simulink model "MPSK_passmodem_v2"  (Simulink 7.6)
settings: Solver=FixedStepDiscrete  SolverMode=SingleTasking  StartTime=0.0  StopTime=1  FixedStep=1/100000  RelTol=1e-3  AbsTol=1e-6
PreLoadFcn:
  | fs=1e5; Ts=1/fs; R=1000; T=1/R; fc=10000; M=8; offset=0;
undefined symbols (not defined in the file): get
libraries: simulink x10, commfilt2 x6, commsink2 x4, simulink_extras x2, commutil2 x2, commchan3 x1, commrandsrc2 x1
settings Model: Creator=amoura  LastModifiedBy=Sílvio
settings DataIOCC: LimitDataPoints=off
settings OptimizationCC: BlockReduction=off  BooleanDataType=off  InitFltsAndDblsToZero=on
settings DebuggingCC: SaveWithParameterizedLinksMsg=none  SignalResolutionControl=TryResolveAllWithWarning  SolverPrmCheckMsg=none  MultiTaskDSMMsg=warning  MultiTaskCondExecSysMsg=none  StrictBusMsg=None
settings HardwareCC: TargetUnknown=on
settings RTWCC: TemplateMakefile=grt_unix.tmf  IncludeERTFirstTime=on
settings GRTTargetCC: TargetFcnLib=ansi_tfl_tmw.mat  ModelReferenceCompliant=off  MatFileLogging=off

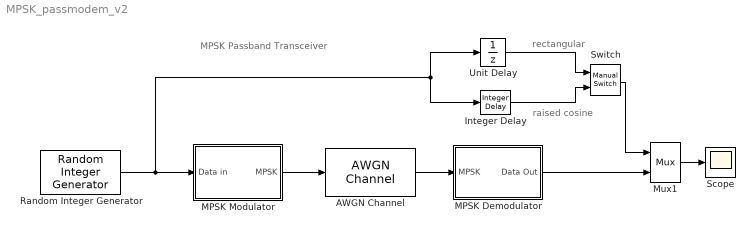
== system MPSK_passmodem_v2 ==
  note: raised cosine
  note: rectangular
  note: MPSK Passband Transceiver
  AWGN Channel : commchan3/AWGN Channel  SystemSampleTime=-1  InputProcessing=Columns as channels (frame based)  seed=67  noiseMode="Signal to noise ratio  (Es/No)"  EbNodB=0  EsNodB=100  SNRdB=10  bitsPerSym=1  Ps=1  Tsym=T  variance=0.1
  Integer Delay : simulink/Discrete/Integer Delay  NumDelays=2*5  vinit=0  samptime=-1
  MPSK Demodulator : Subsystem
  MPSK Modulator : Subsystem
  Mux1 : Mux  Inputs=2
  Random Integer Generator : commrandsrc2/Random Integer Generator  SystemSampleTime=-1  mul=M  seed=96931  Ts=T  frameBased=off  sampPerFrame=100  orient=off  outDataType=double
  Scope : Scope
      settings: TickLabels=on  YMin=-1  YMax=8  DataFormat=Array
  Switch : simulink/Signal Routing/Manual Switch  SystemSampleTime=-1  sw=0  action=0  varsize=off
  Unit Delay : UnitDelay  SampleTime=T
  wires:
  MPSK Modulator/1(MPSK) -> AWGN Channel/1
  Mux1/1 -> Scope/1
  Random Integer Generator/1 -> MPSK Modulator/1(Data in), Unit Delay/1, Integer Delay/1
  MPSK Demodulator/1(Data Out) -> Mux1/2
  AWGN Channel/1 -> MPSK Demodulator/1(MPSK)
  Integer Delay/1 -> Switch/2
  Unit Delay/1 -> Switch/1
  Switch/1 -> Mux1/1

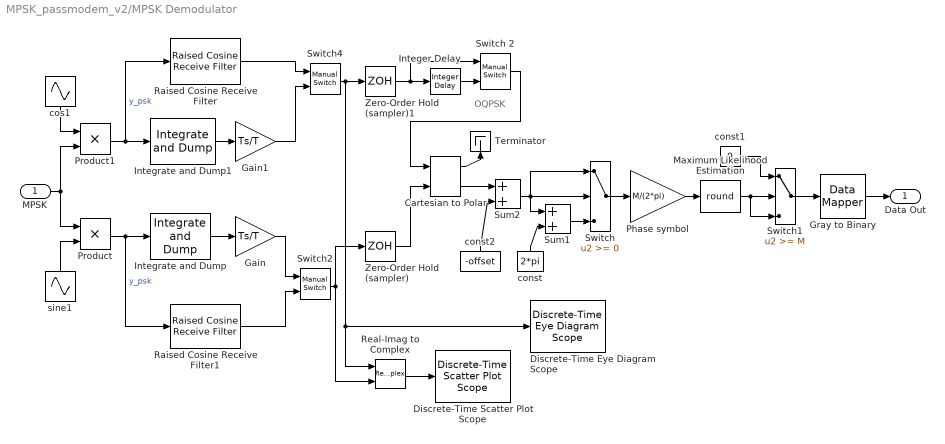
== system MPSK_passmodem_v2/MPSK Demodulator ==
  note: OQPSK
  MPSK : Inport
  Cartesian to Polar : simulink_extras/Transformations/Cartesian to Polar  SystemSampleTime=-1
  Discrete-Time Eye Diagram Scope : commsink2/Discrete-Time Eye Diagram Scope  Tag=EyeDiagram  SystemSampleTime=-1  sampPerSymb=100  offsetEye=0  symbPerTrace=2  numTraces=100  numNewFrames=4  LineStyles=-  LineColors=b  dupPoints=on  fading=on  render=on  AxisGrid=on  yMin=-0.707831262397474  yMax=0.776216891487404  inphaseLabel=In-phase Amplitude  quadratureLabel=Quadrature Amplitude  openScopeAtSimStart=on  dispDiagram=In-phase Only  FrameNumber=off  FigPos=get(0,'defaultfigureposition');  figTitle=Receiver In-Phase Eye Diagram  block_type_=eye  numLinesMax=8
  Discrete-Time Scatter Plot Scope : commsink2/Discrete-Time Scatter Plot Scope  Tag=ScatterPlot  SystemSampleTime=-1  sampPerSymb=fs/R  offsetEye=0  numTraces=40  numNewFrames=10  LineMarkers=.  LineColors=b  fading=on  render=on  AxisGrid=on  xMin=-0.526661007972348  xMax=0.526437343582541  yMin=-0.52656219857096  yMax=0.526536152983929  inphaseLabel=In-phase Amplitude  quadratureLabel=Quadrature Amplitude  openScopeAtSimStart=on  FrameNumber=off  FigPos=get(0,'defaultfigureposition');  figTitle=Receiver Scatter Plot  numLinesMax=8  block_type_=scatter
  Gain : Gain  Gain=Ts/T  SampleTime=Ts  SaturateOnIntegerOverflow=on  OutDataTypeStr=Inherit: Same as input  ParamDataTypeStr=Inherit: Same as input
  Gain1 : Gain  Gain=Ts/T  SampleTime=Ts  SaturateOnIntegerOverflow=on  OutDataTypeStr=Inherit: Same as input  ParamDataTypeStr=Inherit: Same as input
  Gray to Binary : commutil2/Data Mapper  SystemSampleTime=-1  MapMode=Gray to Binary  M=M  MapVec=[0 1 3 2 7 6 4 5]
  Integer Delay : simulink/Discrete/Integer Delay  NumDelays=(T/Ts)/2  vinit=0  samptime=-1
  Integrate and Dump : commfilt2/Integrate and Dump  DialogController=commDDGCreate  DialogControllerArgs=DataTag3  obssamples=T/Ts  offsetsamples=1  nodump=on  roundingMode=Floor  overflowMode=off
  Integrate and Dump1 : commfilt2/Integrate and Dump  DialogController=commDDGCreate  DialogControllerArgs=DataTag4  obssamples=T/Ts  offsetsamples=1  nodump=on  roundingMode=Floor  overflowMode=off
  Maximum Likelihood Estimation : Rounding  Operator=round
  Phase symbol : Gain  Gain=M/(2*pi)  SaturateOnIntegerOverflow=on  OutDataTypeStr=Inherit: Same as input  ParamDataTypeStr=Inherit: Same as input
  Product : Product  SampleTime=1/100000  SaturateOnIntegerOverflow=on  RndMeth=Zero  InputSameDT=on  OutDataTypeStr=Inherit: Same as first input
  Product1 : Product  SampleTime=1/100000  SaturateOnIntegerOverflow=on  RndMeth=Zero  InputSameDT=on  OutDataTypeStr=Inherit: Same as first input
  Raised Cosine Receive Filter : commfilt2/Raised Cosine Receive Filter  DialogController=dspDDGCreate  DialogControllerArgs=DataTag6  SystemSampleTime=-1  filtType=Normal  N=100  D=5  R=0.4  sampMode=Mute  saveAsFlag=0  rateMode=None  downFactor=100  downOffset=0  framing=Enforce single-rate processing  InputProcessing=Columns as channels (frame based)  checkGain=Normalized  filterGain=1  checkCoeff=off  variableName=rcRxFilt  launchFVT=off  roundingMode=Floor  overflowMode=off
  Raised Cosine Receive Filter1 : commfilt2/Raised Cosine Receive Filter  DialogController=dspDDGCreate  DialogControllerArgs=DataTag8  SystemSampleTime=-1  filtType=Normal  N=100  D=5  R=0.4  sampMode=Mute  saveAsFlag=0  rateMode=None  downFactor=100  downOffset=0  framing=Enforce single-rate processing  InputProcessing=Columns as channels (frame based)  checkGain=Normalized  filterGain=1  checkCoeff=off  variableName=rcRxFilt1  launchFVT=off  roundingMode=Floor  overflowMode=off
  Real-Imag to Complex : RealImagToComplex
  Sum1 : Sum  SaturateOnIntegerOverflow=on  InputSameDT=on  OutDataTypeStr=Inherit: Same as first input
  Sum2 : Sum  SaturateOnIntegerOverflow=on  InputSameDT=on  OutDataTypeStr=Inherit: Same as first input
  Switch : Switch  SaturateOnIntegerOverflow=on  InputSameDT=on
  Switch 2 : simulink/Signal Routing/Manual Switch  SystemSampleTime=-1  sw=1  action=0  varsize=off
  Switch1 : Switch  Threshold=M
  Switch2 : simulink/Signal Routing/Manual Switch  SystemSampleTime=-1  sw=1  action=0  varsize=off
  Switch4 : simulink/Signal Routing/Manual Switch  SystemSampleTime=-1  sw=0  action=0  varsize=off
  Terminator : Terminator
  Zero-Order Hold (sampler) : ZeroOrderHold  SampleTime=T
  Zero-Order Hold (sampler)1 : ZeroOrderHold  SampleTime=T
  const : Constant  Value=2*pi
  const1 : Constant  Value=0
  const2 : Constant  Value=-offset
  cos1 : Sin  Frequency=2*pi*fc  Phase=pi/2  SampleTime=0
  sine1 : Sin  Frequency=2*pi*fc  SampleTime=0
  Data Out : Outport
  wires:
  Product/1 -> Raised Cosine Receive Filter1/1, Integrate and Dump/1  "y_psk"
  MPSK/1 -> Product1/2, Product/1
  Integrate and Dump/1 -> Gain/1
  sine1/1 -> Product/2
  Product1/1 -> Integrate and Dump1/1, Raised Cosine Receive Filter/1  "y_psk"
  Integrate and Dump1/1 -> Gain1/1
  cos1/1 -> Product1/1
  Sum1/1 -> Switch/3
  Switch/1 -> Phase symbol/1
  Cartesian to Polar/1 -> Terminator/1
  Phase symbol/1 -> Maximum Likelihood Estimation/1
  Zero-Order Hold (sampler)/1 -> Cartesian to Polar/2
  const/1 -> Sum1/2
  Switch1/1 -> Gray to Binary/1
  Maximum Likelihood Estimation/1 -> Switch1/2, Switch1/3
  const1/1 -> Switch1/1
  Real-Imag to Complex/1 -> Discrete-Time Scatter Plot Scope/1
  Gray to Binary/1 -> Data Out/1
  Sum2/1 -> Switch/2, Switch/1, Sum1/1
  Raised Cosine Receive Filter/1 -> Switch4/1
  Gain1/1 -> Switch4/2
  Switch4/1 -> Zero-Order Hold (sampler)1/1, Discrete-Time Eye Diagram Scope/1, Real-Imag to Complex/1
  Gain/1 -> Switch2/1
  Switch2/1 -> Zero-Order Hold (sampler)/1, Real-Imag to Complex/2
  const2/1 -> Sum2/2
  Cartesian to Polar/2 -> Sum2/1
  Raised Cosine Receive Filter1/1 -> Switch2/2
  Integer Delay/1 -> Switch 2/2
  Zero-Order Hold (sampler)1/1 -> Integer Delay/1, Switch 2/1
  Switch 2/1 -> Cartesian to Polar/1

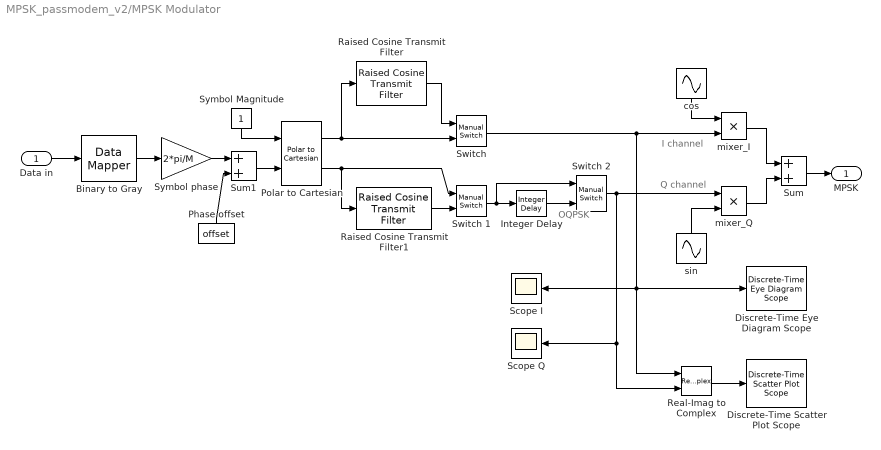
== system MPSK_passmodem_v2/MPSK Modulator ==
  note: I channel
  note: Q channel
  note: OQPSK
  Data in : Inport
  Binary to Gray : commutil2/Data Mapper  SystemSampleTime=-1  MapMode=Binary to Gray  M=M  MapVec=[0 1 3 2 7 6 4 5]
  Discrete-Time Eye Diagram Scope : commsink2/Discrete-Time Eye Diagram Scope  Tag=EyeDiagram  SystemSampleTime=-1  sampPerSymb=100  offsetEye=0  symbPerTrace=2  numTraces=100  numNewFrames=4  LineStyles=-  LineColors=b  dupPoints=on  fading=on  render=on  AxisGrid=on  yMin=-0.141806551380073  yMax=0.145121518302209  inphaseLabel=In-phase Amplitude  quadratureLabel=Quadrature Amplitude  openScopeAtSimStart=on  dispDiagram=In-phase Only  FrameNumber=off  FigPos=get(0,'defaultfigureposition');  figTitle=Transmitter In-Phase Eye Diagram  block_type_=eye  numLinesMax=8
  Discrete-Time Scatter Plot Scope : commsink2/Discrete-Time Scatter Plot Scope  Tag=ScatterPlot  SystemSampleTime=-1  sampPerSymb=fs/R  offsetEye=0  numTraces=40  numNewFrames=10  LineMarkers=.  LineColors=b  fading=on  render=on  AxisGrid=on  xMin=-0.124708902328642  xMax=0.13818390082743  yMin=-0.133971316328163  yMax=0.128921486827909  inphaseLabel=In-phase Amplitude  quadratureLabel=Quadrature Amplitude  openScopeAtSimStart=on  FrameNumber=off  FigPos=get(0,'defaultfigureposition');  figTitle=Transmitter Scatter Plot  numLinesMax=8  block_type_=scatter
  Integer Delay : simulink/Discrete/Integer Delay  NumDelays=(T/Ts)/2  vinit=0  samptime=-1
  Phase offset : Constant  Value=offset  SampleTime=T
  Polar to Cartesian : simulink_extras/Transformations/Polar to Cartesian  SystemSampleTime=-1
  Raised Cosine Transmit Filter : commfilt2/Raised Cosine Transmit Filter  DialogController=dspDDGCreate  DialogControllerArgs=DataTag11  SystemSampleTime=-1  filtType=Square root  D=5  R=0.4  sampMode=Mute  saveAsFlag=0  N=100  framing=Allow multirate processing  checkGain=Normalized  filterGain=1  checkCoeff=off  variableName=rcTxFilt  launchFVT=off  roundingMode=Floor  overflowMode=off
  Raised Cosine Transmit Filter1 : commfilt2/Raised Cosine Transmit Filter  DialogController=dspDDGCreate  DialogControllerArgs=DataTag13  SystemSampleTime=-1  filtType=Square root  D=5  R=0.4  sampMode=Mute  saveAsFlag=0  N=100  framing=Allow multirate processing  checkGain=Normalized  filterGain=1  checkCoeff=off  variableName=rcTxFilt1  launchFVT=off  roundingMode=Floor  overflowMode=off
  Real-Imag to Complex : RealImagToComplex
  Scope I : Scope
      settings: TickLabels=on  TimeRange=0.01  YMin=-2  YMax=2  DataFormat=Array
  Scope Q : Scope
      settings: TickLabels=on  TimeRange=0.01  YMin=-2  YMax=2  SaveName=ScopeData2  DataFormat=Array
  Sum : Sum  SaturateOnIntegerOverflow=on  InputSameDT=on  OutDataTypeStr=Inherit: Same as first input
  Sum1 : Sum  SaturateOnIntegerOverflow=on  InputSameDT=on  OutDataTypeStr=Inherit: Same as first input
  Switch : simulink/Signal Routing/Manual Switch  SystemSampleTime=-1  sw=1  action=0  varsize=off
  Switch 1 : simulink/Signal Routing/Manual Switch  SystemSampleTime=-1  sw=0  action=0  varsize=off
  Switch 2 : simulink/Signal Routing/Manual Switch  SystemSampleTime=-1  sw=1  action=0  varsize=off
  Symbol Magnitude : Constant  SampleTime=T
  Symbol phase : Gain  Gain=2*pi/M  SaturateOnIntegerOverflow=on  OutDataTypeStr=Inherit: Same as input  ParamDataTypeStr=Inherit: Same as input
  cos : Sin  Frequency=2*pi*fc  Phase=pi/2  SampleTime=0
  mixer_I : Product  SampleTime=Ts  SaturateOnIntegerOverflow=on  InputSameDT=on  OutDataTypeStr=Inherit: Same as first input
  mixer_Q : Product  SampleTime=Ts  SaturateOnIntegerOverflow=on  InputSameDT=on  OutDataTypeStr=Inherit: Same as first input
  sin : Sin  Frequency=2*pi*fc  SampleTime=0
  MPSK : Outport
  wires:
  Symbol Magnitude/1 -> Polar to Cartesian/1
  mixer_I/1 -> Sum/1
  mixer_Q/1 -> Sum/2
  sin/1 -> mixer_Q/2
  Binary to Gray/1 -> Symbol phase/1
  Sum/1 -> MPSK/1
  Data in/1 -> Binary to Gray/1
  Polar to Cartesian/1 -> Raised Cosine Transmit Filter/1, Switch/2
  Polar to Cartesian/2 -> Raised Cosine Transmit Filter1/1, Switch 1/1
  cos/1 -> mixer_I/1
  Symbol phase/1 -> Sum1/1
  Phase offset/1 -> Sum1/2
  Sum1/1 -> Polar to Cartesian/2
  Raised Cosine Transmit Filter/1 -> Switch/1
  Switch/1 -> mixer_I/2, Scope I/1, Discrete-Time Eye Diagram Scope/1, Real-Imag to Complex/1
  Raised Cosine Transmit Filter1/1 -> Switch 1/2
  Switch 1/1 -> Switch 2/1, Integer Delay/1
  Integer Delay/1 -> Switch 2/2
  Switch 2/1 -> mixer_Q/1, Scope Q/1, Real-Imag to Complex/2
  Real-Imag to Complex/1 -> Discrete-Time Scatter Plot Scope/1
